simulink model "paper1_inner_loop1"  (Simulink 6.0)
settings: Solver=ode3  StartTime=0.0  StopTime=10.0  FixedStep=0.01  RelTol=1e-3
settings Model: LastModifiedBy=Administrator

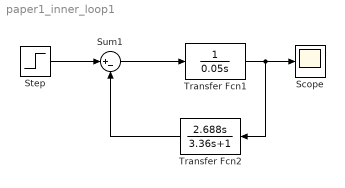
== system paper1_inner_loop1 ==
  Scope : Scope
      settings: SaveName=out  DataFormat=Array
  Step : Step  Time=0  SampleTime=0
  Sum1 : Sum  Inputs=|+-
  Transfer Fcn1 : TransferFcn  Denominator=[0.05 0]
  Transfer Fcn2 : TransferFcn  Orientation=left  Numerator=[2.688 0]  Denominator=[3.36 1]
  wires:
  Transfer Fcn1/1 -> Scope/1, Transfer Fcn2/1
  Sum1/1 -> Transfer Fcn1/1
  Step/1 -> Sum1/1
  Transfer Fcn2/1 -> Sum1/2
